simulink model "secondary_cuk"  (R2020b)
settings: Solver=VariableStepAuto  StartTime=0.0  StopTime=0.6  FixedStep=t_step
undefined symbols (not defined in the file): C1, C2, f_opt, Ion, L1, L2, Lb, Lithium, M, R, R1, R2, R_load, Rb, t_step, Vl
libraries: powerlib x43, powerlib_meascontrol x3, electricdrivelib x1, eePowerMeasurement x1
settings Model: Creator=Chuanyue Li  LastModifiedBy=kjaku
settings DataIOCC: ReturnWorkspaceOutputs=off
settings DebuggingCC: ArithmeticOperatorsInVariantConditions=warning
settings SFSimCC: SimUseLocalCustomCode=off  CustomCodeUndefinedFunction=UseInterfaceOnly
settings RTWCC: RTWUseLocalCustomCode=off

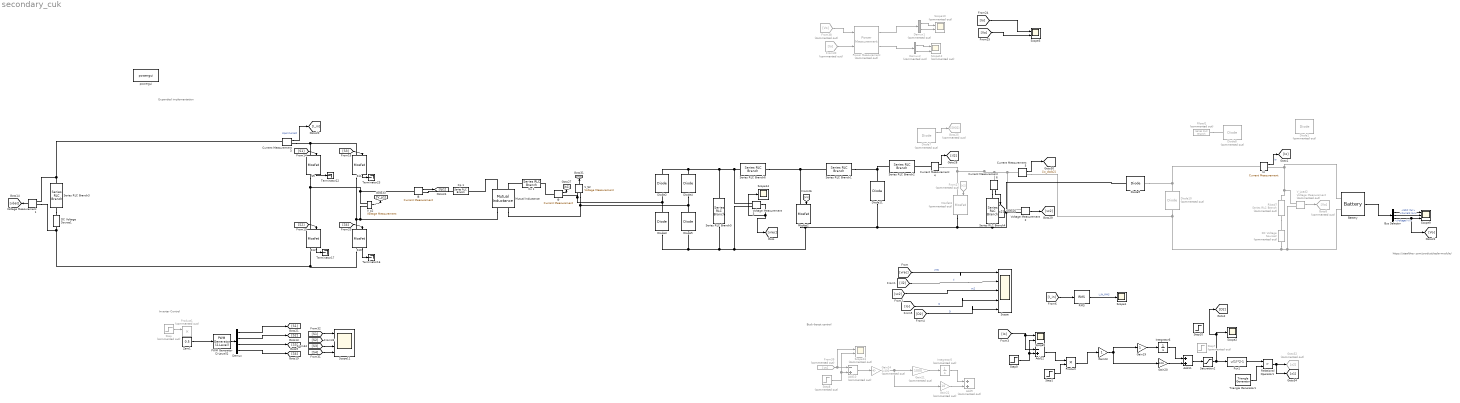
== system secondary_cuk ==
  note: https://stealthev.com/product/tesla-module/
  note: Expanded implementation
  note: Inverter Control
  note: Buck-boost control
  Add10 : Sum  Commented=on  Inputs=-+
  Add11 : Sum
  Add12 : Sum  Inputs=-+
  Add9 : Sum  Commented=on
  Battery : electricdrivelib/Extra Sources/Battery  BatType=Lithium-Ion  ShowTempParam=off  ThermalPreset=no  ShowAgeParam=off  NomV=400  NomQ=230  SOC=50  Batt_Tr=30  PresetModel=on  MaxQ=230  MinV=300  FullV=465.5949  Dis_rate=100  R=0.017391  Normal_OP=208  expZone="[432.1543          11.3]"  current=[6.5 13 32.5]  Units=Time  Tci=20  NomT=20  T2=-30  MaxQ2=4.8  FullV2=7.1  Normal_OP2=5.655  expZone2="[6.58           1]"  Rca=0.6  ti=2000  Dp=0  Neq0=0  Tsim=1e6  Ta1=25  Qeol=5.4*0.9  Reol=0.013333*1.2  Char_age=[2.3478, 3]  Dis_age=[2.3478, 10]  N1=1500  N2=10500  N3=1000  N4=1400  Ta2=45  N5=950
  Bus Selector : BusSelector  OutputSignals=SOC (%),Current (A),Voltage (V)
  Cp 1 : powerlib/Elements/Series RLC Branch  LConnTagsString=__new0  RConnTagsString=__new0  BranchType=C  Resistance=R  Inductance=1e-3  SetiL0=off  InitialCurrent=0  Capacitance=C1  Setx0=off  InitialVoltage=0  Measurements=None
  Cs 1 : powerlib/Elements/Series RLC Branch  LConnTagsString=__new0  RConnTagsString=__new0  BranchType=C  Resistance=R  Inductance=1e-3  SetiL0=off  InitialCurrent=0  Capacitance=C2  Setx0=off  InitialVoltage=0  Measurements=None
  Current Measurement{3..6} (4 alike) : powerlib/Measurements/Current Measurement  PhasorSimulation=off  OutputType=Complex  PSBequivalent=0
  DC Voltage Source1 : powerlib/Electrical Sources/DC Voltage Source  Amplitude=Vl  Measurements=None
  DC Voltage Source2 : powerlib/Electrical Sources/DC Voltage Source  Commented=on  Amplitude=400  Measurements=None
  Demux : Demux
  Demux1 : Demux  Commented=on  Outputs=2
  Demux2 : Demux  Commented=on  Outputs=2
  Diode1 : powerlib/Power Electronics/Diode  Commented=on  Ron=0.001  Lon=0  Vf=0.8  IC=0  UseSnubber=0  Rs=500  Cs=250e-9  Measurements=off
  Diode10 : powerlib/Power Electronics/Diode  Commented=on  Ron=0.001  Lon=0  Vf=0.8  IC=0  UseSnubber=0  Rs=500  Cs=250e-9  Measurements=off
  Diode{2..5,9,11} (6 alike) : powerlib/Power Electronics/Diode  Ron=0.001  Lon=0  Vf=0.8  IC=0  UseSnubber=0  Rs=500  Cs=250e-9  Measurements=off
  Diode7 : powerlib/Power Electronics/Diode  Commented=on  Ron=0.001  Lon=0  Vf=0  IC=0  UseSnubber=0  Rs=500000  Cs=250e-9  Measurements=on
  Diode8 : powerlib/Power Electronics/Diode  Commented=on  Ron=0.001  Lon=0  Vf=0.8  IC=0  UseSnubber=0  Rs=500  Cs=250e-9  Measurements=off
  Fcn1 : Fcn  Expr=u(1)*2-1
  From27 : From  Commented=on  GotoTag=x2
  From30 : From  Commented=on  GotoTag=Io
  From38 : From  Commented=on  GotoTag=Vo
  From39 : From  Commented=on  GotoTag=vc
  Gain19 : Gain
  Gain20 : Gain  Gain=0.01
  Gain21 : Gain  Commented=on  Gain=1000
  Gain22 : Gain  Commented=on  Gain=10
  Gain23 : Gain
  Gain24 : Gain  Commented=on  Gain=1/400
  Goto25 : Goto  Commented=on  GotoTag=iDIO2
  Goto32 : Goto  Commented=on  GotoTag=x2
  Goto8 : Goto  Commented=on  GotoTag=Vo
  I4 : powerlib/Measurements/Current Measurement  PhasorSimulation=off  OutputType=Complex  PSBequivalent=0
  I8 : powerlib/Measurements/Current Measurement  PhasorSimulation=off  OutputType=Complex  PSBequivalent=0
  I9 : powerlib/Measurements/Current Measurement  PhasorSimulation=off  OutputType=Complex  PSBequivalent=0
  Integrator5 : Integrator  Commented=on
  Integrator6 : Integrator
  Mosfet2 : powerlib/Power Electronics/Mosfet  Ron=0.01  Lon=0  Rd=0.01  Vfd=0  IC=0  Rs=1e5  Cs=inf  Measurements=on
  Mosfet3 : powerlib/Power Electronics/Mosfet  Commented=on  Ron=0.01  Lon=0  Rd=0.01  Vfd=0  IC=0  Rs=1e5  Cs=inf  Measurements=on
  Mutual Inductance : powerlib/Elements/Mutual Inductance  LConnTagsString=a|b  RConnTagsString=A|B  TypeOfMutual=Two or three windings with equal mutual terms  NumberOfWindings=3  SelfImpedance1=[R1 L1]  SelfImpedance2=[R2 L2]  ThreeWindings=off  SelfImpedance3=[ 1.1 1.1e-03]  MutualImpedance=[0 M]  InductanceMatrix="[1.0 0.9  0.9 ;  0.9 1.0  0.9;  0.9 0.9 1.0 ] * 1e-3"  ResistanceMatrix="[1.0 0.9  0.9 ;  0.9 1.0  0.9;  0.9 0.9 1.0 ]"  Measurements=None
      settings: AttributesFormatString=\n  SourceProductBaseCode=PS
  PWM Generator (2-Level)2 : powerlib_meascontrol/Pulse & Signal Generators/PWM Generator (2-Level)  ModulatorType=Single-phase full-bridge - Bipolar modulation (4 pulses)  ModulatorMode=Unsynchronized  Fc=f_opt  Pc=90  nF=27  MinMax="[ 0  1 ]"  SamplingTechnique=Natural  ModulatingSignals=off  m=0.8  Freq=60  Phase=0  Ts=0  ShowCarrierOutport=off
  Power Measurement : eePowerMeasurement/Power Measurement  Commented=on  LabelModeActiveChoice=Continuous  F=f_opt*2  K=[0 1]  Ts=0
      settings: SourceProductBaseCode=PS
  Product : Product
  Product1 : Product  Commented=on
  RMS : powerlib_meascontrol/Measurements/RMS  TrueRMS=on  Freq=f_opt  RMSInit=0  Ts=0
  Relational Operator1 : RelationalOperator  Operator=>  OutDataTypeStr=boolean  RndMeth=Zero
  Rload1 : powerlib/Elements/Series RLC Branch  Commented=on  LConnTagsString=__new0  RConnTagsString=__new0  BranchType=L  Resistance=R_load  Inductance=10e-3  SetiL0=off  InitialCurrent=0  Capacitance=100e-6  Setx0=on  InitialVoltage=Vb  Measurements=None
  Rload7 : powerlib/Elements/Series RLC Branch  Commented=on  LConnTagsString=__new0  RConnTagsString=__new0  BranchType=R  Resistance=R_load*0+Rb  Inductance=1e-3  SetiL0=off  InitialCurrent=0  Capacitance=10e-6  Setx0=on  InitialVoltage=300  Measurements=None
  S{9..12} (4 alike) : powerlib/Power Electronics/Mosfet  Ron=0.1  Lon=0  Rd=Rds  Vfd=0  IC=0  Rs=1e5  Cs=inf  Measurements=on
  Saturation2 : Saturate  UpperLimit=0.95  LowerLimit=-1
  Scope : Scope  NumInputPorts=5
  Scope1 : Scope
  Scope10 : Scope  Commented=on  NumInputPorts=2
  Scope11 : Scope  NumInputPorts=4
  Scope12 : Scope  Commented=on  NumInputPorts=2
  Scope13 : Scope  Commented=on  NumInputPorts=2
  Scope14 : Scope
  Scope2 : Scope
  Scope3 : Scope  NumInputPorts=2
  Scope5 : Scope  NumInputPorts=2
  Scope9 : Scope  NumInputPorts=3
  Series RLC Branch1 : powerlib/Elements/Series RLC Branch  LConnTagsString=__new0  RConnTagsString=__new0  BranchType=C  Resistance=1  Inductance=1e-3  SetiL0=off  InitialCurrent=0  Capacitance=10e-6  Setx0=off  InitialVoltage=400  Measurements=None
  Series RLC Branch2 : powerlib/Elements/Series RLC Branch  LConnTagsString=__new0  RConnTagsString=__new0  BranchType=L  Resistance=1  Inductance=Lb  SetiL0=off  InitialCurrent=10  Capacitance=1e-6  Setx0=off  InitialVoltage=0  Measurements=None
  Series RLC Branch3 : powerlib/Elements/Series RLC Branch  LConnTagsString=__new0  RConnTagsString=__new0  BranchType=R  Resistance=Rb  Inductance=Lb  SetiL0=off  InitialCurrent=0  Capacitance=1e-6  Setx0=off  InitialVoltage=0  Measurements=None
  Series RLC Branch4 : powerlib/Elements/Series RLC Branch  LConnTagsString=__new0  RConnTagsString=__new0  BranchType=C  Resistance=1  Inductance=1e-3  SetiL0=off  InitialCurrent=0  Capacitance=100e-6  Setx0=off  InitialVoltage=400  Measurements=None
  Series RLC Branch5 : powerlib/Elements/Series RLC Branch  LConnTagsString=__new0  RConnTagsString=__new0  BranchType=C  Resistance=1  Inductance=1e-3  SetiL0=off  InitialCurrent=0  Capacitance=10e-6  Setx0=off  InitialVoltage=400  Measurements=None
  Series RLC Branch6 : powerlib/Elements/Series RLC Branch  LConnTagsString=__new0  RConnTagsString=__new0  BranchType=L  Resistance=1  Inductance=Lb  SetiL0=off  InitialCurrent=10  Capacitance=1e-6  Setx0=off  InitialVoltage=0  Measurements=None
  Step : Step  Commented=on  Time=0.05  Before=0.3  After=0.35  SampleTime=0
  Step1 : Step  Time=0  SampleTime=0
  Step10 : Step  After=0.6  SampleTime=0
  Step7 : Step  Commented=on  Time=0.3  Before=0.45  After=0.5  SampleTime=0
  Step8 : Step  Commented=on  Time=0.2  Before=410  After=500  SampleTime=0
  Step9 : Step  Before=16  After=6  SampleTime=0
  Terminator{16..17,22..23} (4 alike) : Terminator
  Triangle Generator1 : powerlib_meascontrol/Pulse & Signal Generators/Triangle Generator  Freq=s_fre  Phase=0  Ts=0
  V_Load2 : powerlib/Measurements/Voltage Measurement  Commented=on  PhasorSimulation=off  OutputType=Complex  PSBequivalent=0
  V_S2 : powerlib/Measurements/Voltage Measurement  PhasorSimulation=off  OutputType=Complex  PSBequivalent=0
  V_p2 : powerlib/Measurements/Voltage Measurement  PhasorSimulation=off  OutputType=Complex  PSBequivalent=0
  Voltage Measurement1 : powerlib/Measurements/Voltage Measurement  PhasorSimulation=off  OutputType=Complex  PSBequivalent=0
  Voltage Measurement2 : powerlib/Measurements/Voltage Measurement  PhasorSimulation=off  OutputType=Complex  PSBequivalent=0
  Voltage Measurement3 : powerlib/Measurements/Voltage Measurement  PhasorSimulation=off  OutputType=Complex  PSBequivalent=0
  Zero1 : Constant  Value=0.5  OutDataTypeStr=Inherit: Inherit via back propagation
  powergui : powerlib/powergui  Priority=1  SimulationMode=Continuous  SampleTime=t_step  frequency=60  Iterations=50  frequencyindice=0  Pbase=100e6  ErrMax=1e-4  UnitsV=kV  UnitsW=MW  buscounter=0  FunctionMessages=off  echomessages=off  EnableUseOfTLC=off  CurrentSourceSwitches=off  DisableSnubberDevices=off  DisableRonSwitches=off  DisableVfSwitches=off  DisplayEquations=off  AutomaticDiscreteSolvers=off  SolverType=Tustin/Backward Euler (TBE)  Interpol=off  ExternalGateDelay=off  methode=off  Ts=100  x0status=blocks  SPID=off  SwTol=0  HookPort=off  NonlinearTolerance=1e-4  nMaxIteration=100  ContinueOnMaxIteration=off  RestoreLinks=warning  ResistiveCurrentMeasurement=off  Frange=[0:2:500]  Ylog=off  Xlog=on  ShowGrid=off  save=off  variable=ZData  structure=logsout  ZoomFFT=off  StartTime=0.2  cycles=10  DisplayStyle=2  fundamental=50  FreqAxis=off  MaxFrequency=1000  frequencyindicesteady=1  RmsSteady=1  display=off
  wires:
  Voltage Measurement1/1 -> [vbat]
  Demux/4 -> [S4]
  I4/1 -> [Io]  "Io"
  [S3] -> Scope11/3
  Demux/3 -> [S3]
  [S4] -> S10/1
  I8/1 -> [Ip1]
  Demux/1 -> [S1]
  [S2] -> Scope11/2
  S12/1 -> Terminator17/1
  S11/1 -> Terminator23/1
  [S4] -> Scope11/4
  S10/1 -> Terminator16/1
  Current Measurement3/1 -> [I_in]  "Input Current"
  [S2] -> S12/1
  S9/1 -> Terminator22/1
  [S3] -> S11/1
  V_Load2/1 -> Goto8/1
  V_p2/1 -> [V_p1]
  [S1] -> Scope11/1
  PWM Generator (2-Level)2/1 -> Demux/1
  Demux/2 -> [S2]
  V_S2/1 -> [Vs1]
  Step/1 -> Product1/1
  [S1] -> S9/1
  I9/1 -> [Is1]
  Zero1/1 -> PWM Generator (2-Level)2/1
  [Io] -> Scope3/1
  [Vo] -> Scope3/2
  Battery/1 -> Bus Selector/1
  Bus Selector/1 -> Scope9/1  "<SOC (%)>"
  Bus Selector/2 -> Scope9/2  "<Current (A)>"
  Bus Selector/3 -> [Vo], Scope9/3  "<Voltage (V)>"
  From30/1 -> Power Measurement/2
  From38/1 -> Power Measurement/1
  Power Measurement/1 -> Demux1/1
  Power Measurement/2 -> Demux2/1
  Demux1/1 -> Scope10/1
  Demux1/2 -> Scope10/2
  Demux2/2 -> Scope12/2
  Demux2/1 -> Scope12/1
  [x1] -> Mosfet2/1
  Voltage Measurement2/1 -> [vc2]
  From27/1 -> Mosfet3/1
  Current Measurement6/1 -> [ic2]
  Diode7/1 -> Goto25/1
  Current Measurement4/1 -> [il2]
  Current Measurement5/1 -> [io_dcdc2]
  Gain21/1 -> Integrator5/1
  Saturation2/1 -> Scope2/1, [D2], Fcn1/1
  Step8/1 -> Scope13/2, Add10/2
  Add10/1 -> Gain24/1
  Product/1 -> Gain23/1
  Fcn1/1 -> Relational Operator1/1
  Gain24/1 -> Gain22/1, Gain21/1
  Gain22/1 -> Add9/2
  Integrator5/1 -> Add9/1
  Gain20/1 -> Add11/2
  Add11/1 -> Saturation2/1
  Step9/1 -> Scope5/2, Add12/2
  From39/1 -> Scope13/1, Add10/1
  Gain19/1 -> Integrator6/1
  Relational Operator1/1 -> [x1], Goto32/1
  [Io] -> Add12/1, Scope5/1
  Gain23/1 -> Gain20/1, Gain19/1
  Integrator6/1 -> Add11/1
  Triangle Generator1/1 -> Relational Operator1/2
  Voltage Measurement3/1 -> [vrec], Scope14/1
  Add12/1 -> Product/1
  Step1/1 -> Product/2
  [vrec] -> Scope/1  "vrec"
  [il2] -> Scope/2  "il"
  [vc2] -> Scope/3  "vc2"
  [Io] -> Scope/4  "io"
  [D2] -> Scope/5  "D"
  RMS/1 -> Scope1/1  "I_IN_RMS"
  [I_in] -> RMS/1
  connections:
  S10/RConn1 -- Voltage Measurement1/LConn2 -- DC Voltage Source1/LConn1 -- S12/RConn1
  Series RLC Branch3/LConn1 -- DC Voltage Source1/RConn1
  V_Load2/LConn2 -- Battery/LConn2 -- Current Measurement5/RConn1 -- Diode10/LConn1 -- DC Voltage Source2/LConn1
  Mutual Inductance/RConn1 -- V_p2/LConn2 -- S11/RConn1 -- S10/LConn1
  Diode2/LConn1 -- Diode3/RConn1 -- V_S2/LConn1 -- I9/RConn1
  Current Measurement3/RConn1 -- S11/LConn1 -- S9/LConn1
  V_p2/LConn1 -- S9/RConn1 -- S12/LConn1 -- I8/LConn1
  V_S2/LConn2 -- Diode4/LConn1 -- Diode5/RConn1 -- Mutual Inductance/RConn2
  I8/RConn1 -- Cp 1/RConn1
  Cs 1/LConn1 -- Mutual Inductance/LConn2
  I9/LConn1 -- Cs 1/RConn1
  Mutual Inductance/LConn1 -- Cp 1/LConn1
  Rload7/RConn1 -- DC Voltage Source2/RConn1
  Voltage Measurement1/LConn1 -- Current Measurement3/LConn1 -- Series RLC Branch3/RConn1
  Mosfet3/LConn1 -- Current Measurement4/RConn1 -- Current Measurement5/LConn1 -- Voltage Measurement2/LConn1 -- Current Measurement6/LConn1
  Current Measurement6/RConn1 -- Series RLC Branch4/LConn1
  Rload1/LConn1 -- Diode8/LConn1
  V_Load2/LConn1 -- Battery/LConn1 -- I4/RConn1 -- Rload7/LConn1
  Diode11/LConn1 -- Series RLC Branch2/LConn1 -- Series RLC Branch1/RConn1
  Current Measurement4/LConn1 -- Series RLC Branch2/RConn1
  Diode2/RConn1 -- Voltage Measurement3/LConn1 -- Series RLC Branch6/LConn1 -- Series RLC Branch5/LConn1 -- Diode4/RConn1
  Diode10/RConn1 -- Diode9/RConn1 -- I4/LConn1
  Series RLC Branch4/RConn1 -- Diode9/LConn1 -- Voltage Measurement2/LConn2 -- Mosfet2/RConn1 -- Voltage Measurement3/LConn2 -- Series RLC Branch5/RConn1 -- Diode3/LConn1 -- Diode5/LConn1 -- Diode11/RConn1 -- Mosfet3/RConn1
  Series RLC Branch6/RConn1 -- Series RLC Branch1/LConn1 -- Mosfet2/LConn1
